simulink model "XC_org"  (Simulink 10.0)
settings: Solver=ode45  StartTime=0.0  StopTime=1000  RelTol=1e-3  EnableMultiTasking=on
settings Model: Creator=Administrator  LastModifiedBy=annonymous
settings DataIOCC: LimitDataPoints=on
settings OptimizationCC: ExpressionDepthLimit=2147483647
settings DebuggingCC: SolverPrmCheckMsg=warning  StateNameClashWarn=warning
settings GRTTargetCC: GeneratePreprocessorConditionals=Disable all  CombineOutputUpdateFcns=on  GRTInterface=off
settings ConfigComp: CovExternalEMLEnable=off

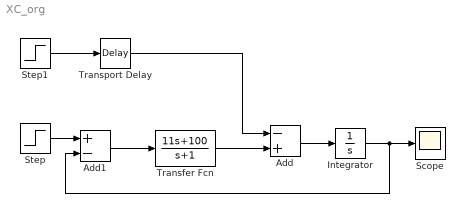
== system XC_org ==
  Add : Sum  Inputs=-+
  Add1 : Sum  Inputs=+-
  Integrator : Integrator
  Scope : Scope
  Step : Step  SampleTime=0
  Step1 : Step  SampleTime=0
  Transfer Fcn : TransferFcn  Numerator=[11 100]  Denominator=[1 1]
  Transport Delay : TransportDelay  DelayTime=0.3
  wires:
  Step1/1 -> Transport Delay/1
  Transport Delay/1 -> Add/1
  Transfer Fcn/1 -> Add/2
  Add/1 -> Integrator/1
  Integrator/1 -> Add1/2, Scope/1
  Step/1 -> Add1/1
  Add1/1 -> Transfer Fcn/1
